simulink model "week3prob1"  (R2020a)
settings: Solver=VariableStepAuto  StartTime=0.0  StopTime=10.0  RelTol=1e-3
settings Model: Creator=Admin  LastModifiedBy=Admin

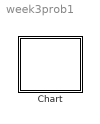
== system week3prob1 ==
  Chart : Stateflow chart  TreatAsAtomicUnit=on

== stateflow chart week3prob1/Chart ==
  state got_0
  state got_nickel
  state got_dime
  (default) -> got_0
  got_0 -> got_nickel [order 1] : [coin == 1]{soda = 0;}
  got_nickel -> got_0 [order 1] : [coin == 2]{soda = 1;}
  got_dime -> got_0 [order 1] : [coin == 1]{soda = 1;}
  got_0 -> got_dime [order 2] : [coin == 2]{soda = 0;}
  got_nickel -> got_dime [order 2] : [coin == 1]{soda = 0;}
  got_dime -> got_nickel [order 2] : [coin == 2]{soda = 1;}
